simulink model "relay"  (R2024b)
settings: Solver=VariableStepAuto  StartTime=0.0  StopTime=0.2  RelTol=1e-3
libraries: spsUniversalBridgeLib x1, powerlib_extras x1, spsPermanentMagnetSynchronousMachineLib x1, spsDCVoltageSourceLib x1, spsabctodq0Lib x1, sps_lib x1

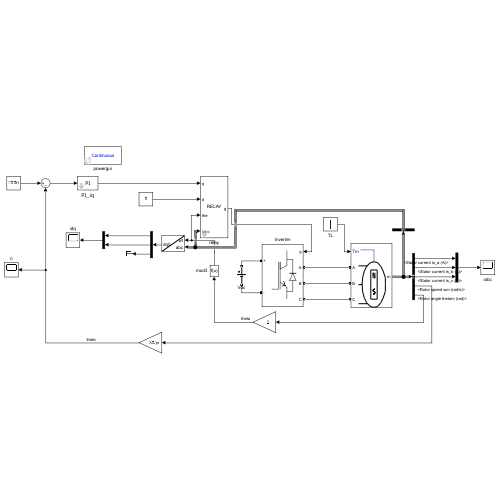
[thumbnail: Simulink's stored preview of the top-level diagram]
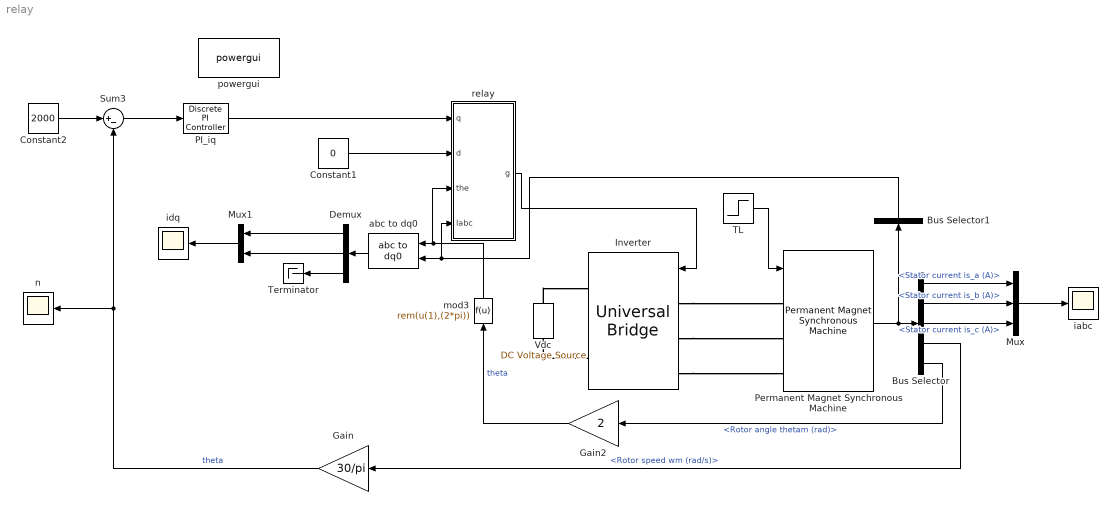
== system relay ==
  Bus Selector : BusSelector  OutputSignals=Stator current is_a (A),Stator current is_b (A),Stator current is_c (A),Rotor speed wm (rad/s),Rotor angle thetam (rad)
  Bus Selector1 : BusSelector  OutputSignals=Stator current is_a (A),Stator current is_b (A),Stator current is_c (A)  OutputAsBus=on
  Constant1 : Constant  Value=0
  Constant2 : Constant  Value=2000
  Demux : Demux  Outputs=3
  Gain : Gain  Gain=30/pi
  Gain2 : Gain  Gain=2
  Inverter : spsUniversalBridgeLib/Universal Bridge  Arms=3  SnubberResistance=1e5  SnubberCapacitance=inf  Device=IGBT / Diodes  Ron=1e-3  Lon=0  ForwardVoltages="[  0  0  ]"  ForwardVoltage=0  GTOparameters=[ 10e-6 , 20e-6 ]  IGBTparameters=[ 1e-6 , 2e-6 ]  Measurements=None  Measurements_2=None  converterType=Rectifier
  Mux : Mux  Inputs=3
  Mux1 : Mux  Inputs=2
  PI_iq : powerlib_extras/Discrete  Control Blocks/Discrete PI Controller  Kp=0.05  Ki=10  Par_Limits=[10 -10]  Init=0  Ts=200e-6
  Permanent Magnet Synchronous Machine : spsPermanentMagnetSynchronousMachineLib/Permanent Magnet Synchronous Machine  NbPhases=3  FluxDistribution=Sinusoidal  RotorType=Salient-pole  MechanicalLoad=Torque Tm  PresetModel="01:  0.8 Nm 300 Vdc 3000 RPM - 0.8 Nm"  ShowDetailedParameters=on  MeasurementBus=off  Resistance=18.7  Inductance=8.5e-3  dqInductances=[0.02547 0.02816]  La=0.000395  MachineConstant=Flux linkage established by magnets (V.s)  Flux=0.1716  VoltageCst=62.2496  TorqueCst=0.5148  Flat=120  Mechanical=[2.26e-05 1.349e-05 2 0]  PolePairs=2  InitialConditions=[0,0, 0,0]  InitialConditions5ph=[0 0 0 0 0 0]  RefAngle=Aligned with phase A axis (original Park)  IterativeDiscreteModel=Trapezoidal non iterative  TsBlock=-1  TsPowergui=0
  Sum3 : Sum  Inputs=|+-
  TL : Step  Time=0.1  After=2  SampleTime=0
  Terminator : Terminator
  Vdc : spsDCVoltageSourceLib/DC Voltage Source  Amplitude=311  Measurements=None
  abc to dq0 : spsabctodq0Lib/abc to dq0  Alignment=Aligned with phase A axis
  iabc : Scope
  idq : Scope
  mod3 : Fcn  Expr=rem(u(1),(2*pi))
  n : Scope
  powergui : sps_lib/powergui  Priority=1  SimulationMode=Continuous  SampleTime=10e-6  frequency=60  Iterations=50  frequencyindice=0  Pbase=100e6  ErrMax=1e-4  UnitsV=kV  UnitsW=MW  buscounter=0  FunctionMessages=off  echomessages=off  EnableUseOfTLC=off  CurrentSourceSwitches=off  DisableSnubberDevices=off  DisableRonSwitches=off  DisableVfSwitches=off  DisplayEquations=off  AutomaticDiscreteSolvers=off  SolverType=Tustin/Backward Euler (TBE)  Interpol=off  ExternalGateDelay=off  methode=off  Ts=100  x0status=blocks  SPID=on  SwTol=0  HookPort=off  NonlinearTolerance=1e-4  nMaxIteration=100  ContinueOnMaxIteration=off  RestoreLinks=warning  ResistiveCurrentMeasurement=off  Frange=[0:2:500]  Ylog=off  Xlog=on  ShowGrid=off  save=off  variable=ZData  structure=0  ZoomFFT=off  StartTime=0.0  cycles=1  DisplayStyle=1  fundamental=60  FreqAxis=off  MaxFrequency=1000  frequencyindicesteady=1  RmsSteady=1  display=off
  relay : Subsystem  mask{thre=0.05}
      mask prompts: thre "threshold"
  wires:
  TL/1 -> Permanent Magnet Synchronous Machine/1
  Permanent Magnet Synchronous Machine/1 -> Bus Selector1/1, Bus Selector/1
  Bus Selector/1 -> Mux/1  "<Stator current is_a (A)>"
  Bus Selector/2 -> Mux/2  "<Stator current is_b (A)>"
  Bus Selector/3 -> Mux/3  "<Stator current is_c (A)>"
  relay/1(g) -> Inverter/1
  Bus Selector/4 -> Gain/1  "<Rotor speed wm (rad/s)>"
  Gain/1 -> Sum3/2, n/1  "theta"
  Mux/1 -> iabc/1
  abc to dq0/1 -> Demux/1
  PI_iq/1 -> relay/1(q)
  Demux/1 -> Mux1/1
  Demux/3 -> Terminator/1
  Sum3/1 -> PI_iq/1
  Constant2/1 -> Sum3/1
  Mux1/1 -> idq/1
  Bus Selector1/1 -> abc to dq0/1, relay/4(Iabc)
  mod3/1 -> relay/3(the), abc to dq0/2
  Gain2/1 -> mod3/1  "theta"
  Bus Selector/5 -> Gain2/1  "<Rotor angle thetam (rad)>"
  Demux/2 -> Mux1/2
  Constant1/1 -> relay/2(d)
  connections:
  Inverter/LConn1 -- Permanent Magnet Synchronous Machine/LConn1
  Inverter/LConn2 -- Permanent Magnet Synchronous Machine/LConn2
  Inverter/LConn3 -- Permanent Magnet Synchronous Machine/LConn3
  Vdc/RConn1 -- Inverter/RConn1
  Inverter/RConn2 -- Vdc/LConn1

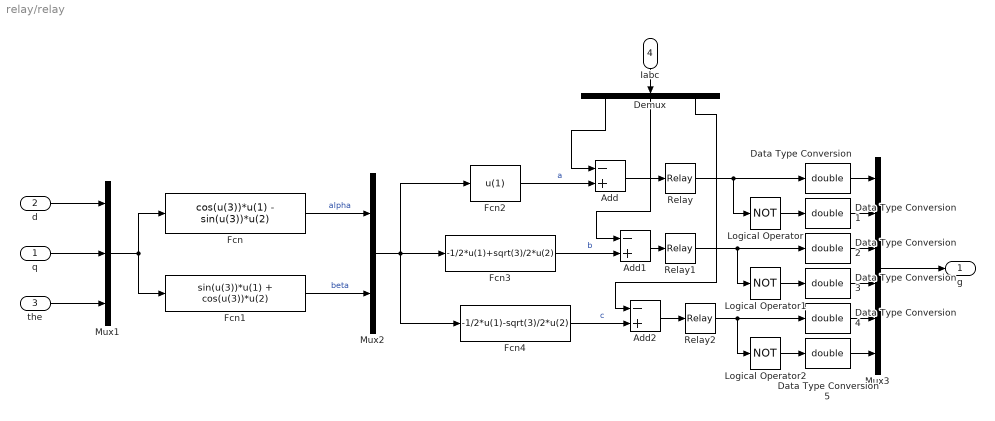
== system relay/relay ==
  q : Inport
  d : Inport  Port=2
  the : Inport  Port=3
  Iabc : Inport  Port=4
  Add : Sum  Inputs=-+
  Add1 : Sum  Inputs=-+
  Add2 : Sum  Inputs=-+
  Data Type Conversion{,1..5} (6 alike) : DataTypeConversion  OutDataTypeStr=double  SaturateOnIntegerOverflow=off  RndMeth=Floor
  Demux : Demux  Outputs=3
  Fcn : Fcn  Expr=cos(u(3))*u(1) - sin(u(3))*u(2)
  Fcn1 : Fcn  Expr=sin(u(3))*u(1) + cos(u(3))*u(2)
  Fcn2 : Fcn  Expr=u(1)
  Fcn3 : Fcn  Expr=-1/2*u(1)+sqrt(3)/2*u(2)
  Fcn4 : Fcn  Expr=-1/2*u(1)-sqrt(3)/2*u(2)
  Logical Operator : Logic  Operator=NOT  AllPortsSameDT=off  OutDataTypeStr=boolean
  Logical Operator1 : Logic  Operator=NOT  AllPortsSameDT=off  OutDataTypeStr=boolean
  Logical Operator2 : Logic  Operator=NOT  AllPortsSameDT=off  OutDataTypeStr=boolean
  Mux1 : Mux  Inputs=3
  Mux2 : Mux  Inputs=2
  Mux3 : Mux  Inputs=6
  Relay : Relay  OnSwitchValue=thre  OffSwitchValue=-thre
  Relay1 : Relay  OnSwitchValue=thre  OffSwitchValue=-thre
  Relay2 : Relay  OnSwitchValue=thre  OffSwitchValue=-thre
  g : Outport
  wires:
  q/1 -> Mux1/2
  Fcn/1 -> Mux2/1  "alpha"
  d/1 -> Mux1/1
  Fcn1/1 -> Mux2/2  "beta"
  Mux1/1 -> Fcn/1, Fcn1/1
  the/1 -> Mux1/3
  Mux2/1 -> Fcn2/1, Fcn4/1, Fcn3/1
  Iabc/1 -> Demux/1
  Fcn2/1 -> Add/2  "a"
  Demux/1 -> Add/1
  Add/1 -> Relay/1
  Relay/1 -> Data Type Conversion/1, Logical Operator/1
  Fcn3/1 -> Add1/2  "b"
  Demux/2 -> Add1/1
  Add1/1 -> Relay1/1
  Relay1/1 -> Data Type Conversion2/1, Logical Operator1/1
  Fcn4/1 -> Add2/2  "c"
  Demux/3 -> Add2/1
  Add2/1 -> Relay2/1
  Relay2/1 -> Data Type Conversion4/1, Logical Operator2/1
  Mux3/1 -> g/1
  Data Type Conversion/1 -> Mux3/1
  Logical Operator/1 -> Data Type Conversion1/1
  Data Type Conversion1/1 -> Mux3/2
  Data Type Conversion2/1 -> Mux3/3
  Logical Operator1/1 -> Data Type Conversion3/1
  Data Type Conversion3/1 -> Mux3/4
  Data Type Conversion4/1 -> Mux3/5
  Logical Operator2/1 -> Data Type Conversion5/1
  Data Type Conversion5/1 -> Mux3/6
